simulink model "ur10_NN_v1"  (R2022b)
settings: Solver=ode4  StartTime=0.0  StopTime=5  FixedStep=0.01  MaxStep=0.1  RelTol=1e-2  AbsTol=1e-2
model workspace (MAT data in the model file):
  jointLimits = [-2.94087978961  2.94087978961; -2.50454747661  0.759218224618; -2.94087978961  2.94087978961; -2.15548162621  1.3962634016; -5.06145483078  5.06145483078; -1.53588974176  2.40855436775; -3.99680398707  3.99680398707; 0  0.025; 0  0.025; -2.94087978961  2.94087978961; -2.50454747661  0.759218224618; -2.94087978961  2.94087978961; -2.15548162621  1.3962634016; -5.06145483078  5.06145483078; -1.53588974176  2.40855436775; -3.99680398707  3.99680398707; 0  0.025; 0  0.025]
  q_points = [-0.521158884693  0.491931392418; -0.226045107026  -0.192139666701; -0.000470673510356  -0.00321781893086; 0.204187486975  0.0825184830426; -0.516935337839  0.505690245866; 0.0199734933983  0.0998802945608]
undefined symbols (not defined in the file): cbf_parms, obstacle, replay_rate, ur10
libraries: robotmaniplib x29, neural x27, robotcorelib x10
(part 1 of 2)
settings Model: PauseTimes=3.1  PacingRate=0.220000  Creator=The MathWorks, Inc.  LastModifiedBy=14244039
settings SolverCC: AlgebraicLoopSolver=TrustRegion
settings DebuggingCC: UnconnectedInputMsg=warning  UnconnectedOutputMsg=warning  UnconnectedLineMsg=warning  SFMachineParentedDataDiag=warning
settings ModelReferenceCC: EnableRefExpFcnMdlSchedulingChecks=on
settings RTWCC: DLArmComputeVersion=19.05

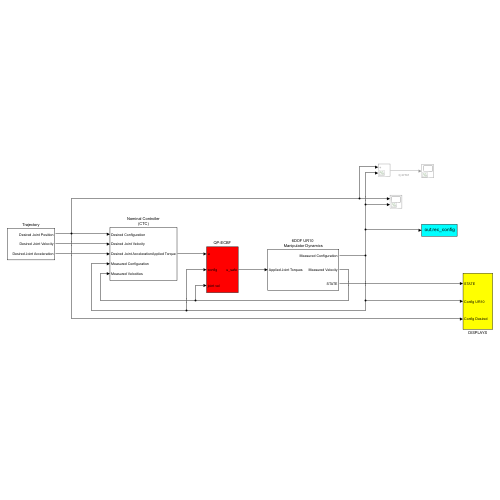
[thumbnail: Simulink's stored preview of the top-level diagram]
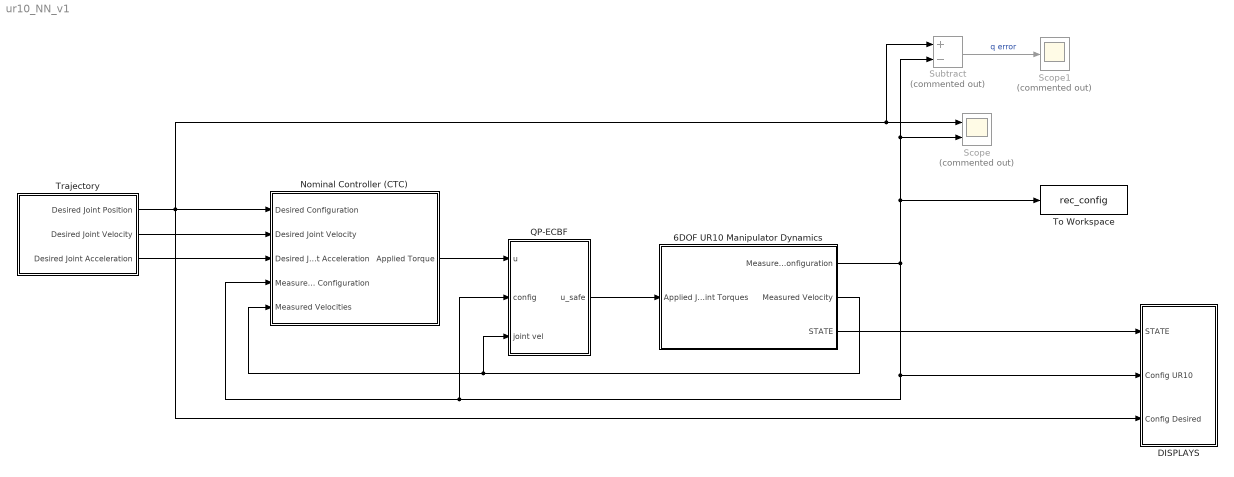
== system ur10_NN_v1 ==
  6DOF UR10 Manipulator Dynamics : Subsystem
  DISPLAYS : Subsystem
  Nominal Controller (CTC) : Subsystem
  QP-ECBF : Subsystem
  Scope : Scope  Commented=on  NumInputPorts=2
  Scope1 : Scope  Commented=on
  Subtract : Sum  Commented=on  Inputs=+-
  To Workspace : ToWorkspace  VariableName=rec_config  SampleTime=replay_rate
  Trajectory : Subsystem
  wires:
  6DOF UR10 Manipulator Dynamics/1(Measured Configuration) -> Subtract/2, Scope/2, To Workspace/1, QP-ECBF/2(config), Nominal Controller (CTC)/4(Measured Configuration), DISPLAYS/2(Config UR10)
  6DOF UR10 Manipulator Dynamics/2(Measured Velocity) -> QP-ECBF/3(joint vel), Nominal Controller (CTC)/5(Measured Velocities)
  Nominal Controller (CTC)/1(Applied Torque) -> QP-ECBF/1(u)
  Subtract/1 -> Scope1/1  "q error"
  QP-ECBF/1(u_safe) -> 6DOF UR10 Manipulator Dynamics/1(Applied Joint Torques)
  6DOF UR10 Manipulator Dynamics/3(STATE) -> DISPLAYS/1(STATE)
  Trajectory/1(Desired Joint Position) -> DISPLAYS/3(Config Desired), Subtract/1, Scope/1, Nominal Controller (CTC)/1(Desired Configuration)
  Trajectory/2(Desired Joint Velocity) -> Nominal Controller (CTC)/2(Desired Joint Velocity)
  Trajectory/3(Desired Joint Acceleration) -> Nominal Controller (CTC)/3(Desired Joint Acceleration)

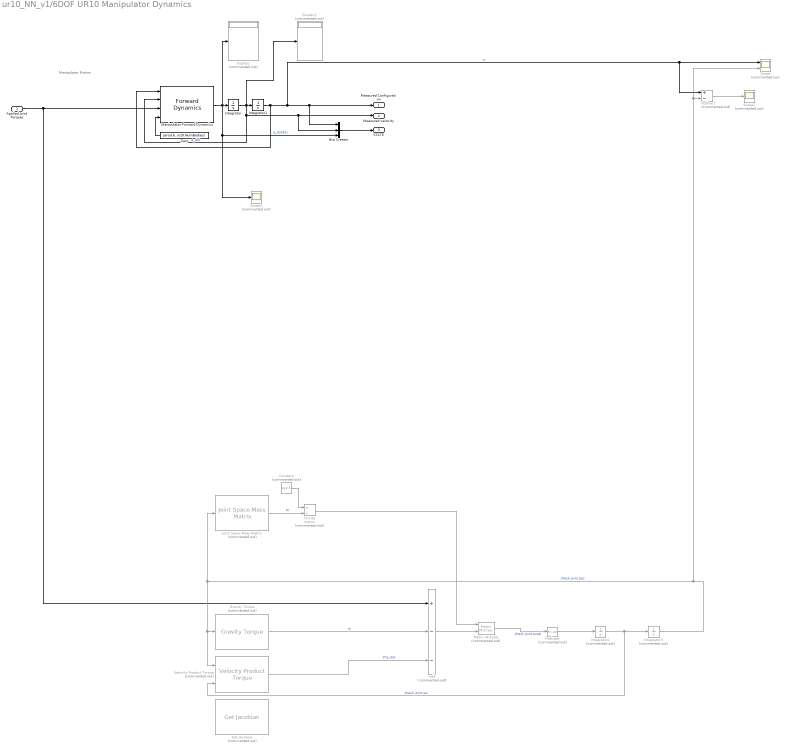
== system ur10_NN_v1/6DOF UR10 Manipulator Dynamics ==
  note: Manipulator Motion
  Applied Joint Torques : Inport
  Add : Sum  Commented=on  Inputs=+--
  Bus Creator : BusCreator  Inputs=3
  Constant : Constant  Commented=on  Value=eye(6)
  Display : Display  Commented=on
  Display1 : Display  Commented=on
  Divide : Product  Commented=on  Inputs=*/  Multiplication=Matrix(*)
  Get Jacobian : robotmaniplib/Get Jacobian  Commented=on  RigidBodyTree=ur10  EndEffector=tool0  SimulateUsing=Interpreted execution
  Gravity Torque : robotmaniplib/Gravity Torque  Commented=on  RigidBodyTree=ur10  SimulateUsing=Interpreted execution
  Integrator : Integrator  InitialCondition=[0 0 0 0 0 0]  UpperSaturationLimit=1000  LowerSaturationLimit=-1000
  Integrator1 : Integrator  InitialCondition=[0 0 0 0 0 0]  UpperSaturationLimit=jointLimits(:,2)  LowerSaturationLimit=jointLimits(:,1)
  Integrator2 : Integrator  Commented=on  InitialCondition=[0 0 0 0 0 0]'
  Integrator3 : Integrator  Commented=on  InitialCondition=[0 0 0 0 0 0]'
  Joint Space Mass Matrix : robotmaniplib/Joint Space Mass Matrix  Commented=on  RigidBodyTree=ur10  SimulateUsing=Interpreted execution
  Manipulator Forward Dynamics : robotmaniplib/Forward Dynamics  RigidBodyTree=ur10  SimulateUsing=Interpreted execution
  Matrix Multiply : Product  Commented=on  Multiplication=Matrix(*)
  Reshape : Reshape  Commented=on
  Scope : Scope  Commented=on  NumInputPorts=2
  Scope1 : Scope  Commented=on
  Scope2 : Scope  Commented=on
  Subtract : Sum  Commented=on  Inputs=+-
  Velocity Product Torque : robotmaniplib/Velocity Product Torque  Commented=on  RigidBodyTree=ur10  SimulateUsing=Interpreted execution
  Zero : Constant  Value=zeros(6, ur10.NumBodies)  OutDataTypeStr=Inherit: Inherit via back propagation
  Measured Configuration : Outport  VectorParamsAs1DForOutWhenUnconnected=off
  Measured Velocity : Outport  Port=2  VectorParamsAs1DForOutWhenUnconnected=off
  STATE : Outport  Port=3  VectorParamsAs1DForOutWhenUnconnected=off
  wires:
  Zero/1 -> Manipulator Forward Dynamics/4
  Integrator/1 -> Display1/1, Manipulator Forward Dynamics/2, Measured Velocity/1, Bus Creator/2, Integrator1/1  "q_dot"
  Applied Joint Torques/1 -> Add/1, Manipulator Forward Dynamics/3
  Integrator1/1 -> Manipulator Forward Dynamics/1, Subtract/1, Scope/1, Measured Configuration/1, Bus Creator/1  "q"
  Manipulator Forward Dynamics/1 -> Scope2/1, Bus Creator/3, Display/1, Integrator/1  "q_dotdot"
  Subtract/1 -> Scope1/1
  Integrator2/1 -> Velocity Product Torque/2, Integrator3/1  "check joint vel"
  Velocity Product Torque/1 -> Add/3  "C*q_dot"
  Gravity Torque/1 -> Add/2  "G"
  Joint Space Mass Matrix/1 -> Divide/2  "M"
  Integrator3/1 -> Subtract/2, Scope/2, Joint Space Mass Matrix/1, Gravity Torque/1, Velocity Product Torque/1  "check joint pos"
  Add/1 -> Matrix Multiply/2
  Divide/1 -> Matrix Multiply/1
  Constant/1 -> Divide/1
  Matrix Multiply/1 -> Reshape/1  "check joint accel"
  Reshape/1 -> Integrator2/1
  Bus Creator/1 -> STATE/1

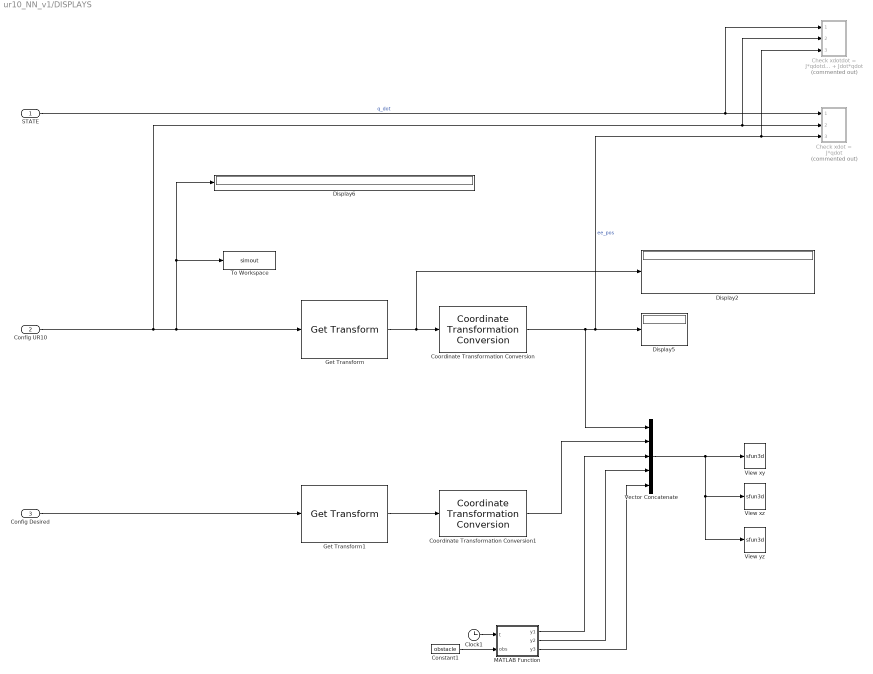
== system ur10_NN_v1/DISPLAYS ==
  STATE : Inport
  Config UR10 : Inport  Port=2
  Config Desired : Inport  Port=3
  Check xdot = J*qdot : Subsystem  Commented=on
  Check xdotdot = J*qdotdot + Jdot*qdot : Subsystem  Commented=on
  Clock1 : Clock
  Constant1 : Constant  Value=obstacle
  Coordinate Transformation Conversion : robotcorelib/Coordinate Transformation Conversion  InputRepresentation=Homogeneous Transformation  InputEulerSequence=ZYX  ShowTrVecInputPort=on  OutputRepresentation=Translation Vector  OutputEulerSequence=ZYX  ShowTrVecOutputPort=on  SimulateUsing=Interpreted execution
  Coordinate Transformation Conversion1 : robotcorelib/Coordinate Transformation Conversion  InputRepresentation=Homogeneous Transformation  InputEulerSequence=ZYX  ShowTrVecInputPort=on  OutputRepresentation=Translation Vector  OutputEulerSequence=ZYX  ShowTrVecOutputPort=on  SimulateUsing=Interpreted execution
  Display2 : Display
  Display5 : Display
  Display6 : Display
  Get Transform : robotmaniplib/Get Transform  RigidBodyTree=ur10  SourceBody=tool0  TargetBody=world  SimulateUsing=Interpreted execution
  Get Transform1 : robotmaniplib/Get Transform  RigidBodyTree=ur10  SourceBody=tool0  TargetBody=world  SimulateUsing=Interpreted execution
  MATLAB Function : MATLAB Function  TreatAsAtomicUnit=on
  To Workspace : ToWorkspace  VariableName=simout  SampleTime=-1
      settings: MaxDataPoints=1  Save2DSignal=2-D array (concatenate along first dimension)
  Vector Concatenate : Concatenate  NumInputs=5
  View xy : S-Function  LoadFcn=if exist('sfun3d','file'), sfun3d([],[],[],'LoadBlock'); end  FunctionName=sfun3d  Parameters=ax,T,np,cp,gd,ls,mk,mx,hd,tb  SFunctionDeploymentMode=off  EnableBusSupport=off  mask(3D Graph){np=5, ax=[-1.5 1.5 -1.5 1.5 -1.5 1.5], mx=1e4, T=0.1, cp=[0         0   25.9808], gd=on, hd=on, tb=on, ls=-, mk=none}
      mask prompts: np "Number of moving points (lines)"; ax "Range: [xmin xmax  ymin ymax zmin zmax]"; mx "Max number of points in each line"; T "Sampling Time"; cp "Camera position (use [0 0 1] for 2D XY view)"; gd "Grid (on|off)"; hd "HeadMarkers (on|off)"; tb "Toolbar (on|off)"; ls "LineStyle"; mk "LineMarker"
      mask help:
      | This block plots the position of several points in the XYZ space. The input contains the coordinates of all the points (x1,y1,z1,x2,y2,z2,...).
      | The number of moving points (lines), the XYZ ranges, sampling time, camera position, and grid (among other things) can be set as mask parameters.
      settings: CopyFcn=if exist('sfun3d','file'), sfun3d([],[],[],'CopyBlock'); end  DeleteFcn=if exist('sfun3d','file'), sfun3d([],[],[],'DeleteBlock'); end  NameChangeFcn=if exist('sfun3d','file'), sfun3d([],[],[],'NameChange'); end
      mask Help:
      | This block plots the position of several points in the XYZ space. The input contains the coordinates of all the points (x1,y1,z1,x2,y2,z2,...).
      | The number of moving points (lines), the XYZ ranges, sampling time, camera position, and grid (among other things) can be set as mask parameters.
      mask TypeOptions ls: - | -- | : | -. | none
      mask TypeOptions mk: none | . | + | o | * | x | square | diamond | v | ^ | > | < | pentagram | hexagram
      mask Display: plot([.05 .95 .95 .05 .05],[.45 .45 .95 .95 .45], 0.5+cos(0:0.1:2*pi)*0.3,0.7+sin(0:0.1:2*pi)*0.2)
  View xz : S-Function  LoadFcn=if exist('sfun3d','file'), sfun3d([],[],[],'LoadBlock'); end  FunctionName=sfun3d  Parameters=ax,T,np,cp,gd,ls,mk,mx,hd,tb  SFunctionDeploymentMode=off  EnableBusSupport=off  mask(3D Graph){np=5, ax=[-1.5 1.5 -1.5 1.5 -1.5 1.5], mx=1e4, T=0.1, cp=[0  -25.9808         0], gd=on, hd=on, tb=on, ls=-, mk=none}
      mask prompts: np "Number of moving points (lines)"; ax "Range: [xmin xmax  ymin ymax zmin zmax]"; mx "Max number of points in each line"; T "Sampling Time"; cp "Camera position (use [0 0 1] for 2D XY view)"; gd "Grid (on|off)"; hd "HeadMarkers (on|off)"; tb "Toolbar (on|off)"; ls "LineStyle"; mk "LineMarker"
      mask help:
      | This block plots the position of several points in the XYZ space. The input contains the coordinates of all the points (x1,y1,z1,x2,y2,z2,...).
      | The number of moving points (lines), the XYZ ranges, sampling time, camera position, and grid (among other things) can be set as mask parameters.
      settings: CopyFcn=if exist('sfun3d','file'), sfun3d([],[],[],'CopyBlock'); end  DeleteFcn=if exist('sfun3d','file'), sfun3d([],[],[],'DeleteBlock'); end  NameChangeFcn=if exist('sfun3d','file'), sfun3d([],[],[],'NameChange'); end
      mask Help:
      | This block plots the position of several points in the XYZ space. The input contains the coordinates of all the points (x1,y1,z1,x2,y2,z2,...).
      | The number of moving points (lines), the XYZ ranges, sampling time, camera position, and grid (among other things) can be set as mask parameters.
      mask TypeOptions ls: - | -- | : | -. | none
      mask TypeOptions mk: none | . | + | o | * | x | square | diamond | v | ^ | > | < | pentagram | hexagram
      mask Display: plot([.05 .95 .95 .05 .05],[.45 .45 .95 .95 .45], 0.5+cos(0:0.1:2*pi)*0.3,0.7+sin(0:0.1:2*pi)*0.2)
  View yz : S-Function  LoadFcn=if exist('sfun3d','file'), sfun3d([],[],[],'LoadBlock'); end  FunctionName=sfun3d  Parameters=ax,T,np,cp,gd,ls,mk,mx,hd,tb  SFunctionDeploymentMode=off  EnableBusSupport=off  mask(3D Graph){np=5, ax=[-1.5 1.5 -0.1 1.5 -1.5 1.5], mx=1e4, T=0.1, cp=[ 25.6976    0.8076   -0.1347], gd=on, hd=on, tb=on, ls=-, mk=none}
      mask prompts: np "Number of moving points (lines)"; ax "Range: [xmin xmax  ymin ymax zmin zmax]"; mx "Max number of points in each line"; T "Sampling Time"; cp "Camera position (use [0 0 1] for 2D XY view)"; gd "Grid (on|off)"; hd "HeadMarkers (on|off)"; tb "Toolbar (on|off)"; ls "LineStyle"; mk "LineMarker"
      mask help:
      | This block plots the position of several points in the XYZ space. The input contains the coordinates of all the points (x1,y1,z1,x2,y2,z2,...).
      | The number of moving points (lines), the XYZ ranges, sampling time, camera position, and grid (among other things) can be set as mask parameters.
      settings: CopyFcn=if exist('sfun3d','file'), sfun3d([],[],[],'CopyBlock'); end  DeleteFcn=if exist('sfun3d','file'), sfun3d([],[],[],'DeleteBlock'); end  NameChangeFcn=if exist('sfun3d','file'), sfun3d([],[],[],'NameChange'); end
      mask Help:
      | This block plots the position of several points in the XYZ space. The input contains the coordinates of all the points (x1,y1,z1,x2,y2,z2,...).
      | The number of moving points (lines), the XYZ ranges, sampling time, camera position, and grid (among other things) can be set as mask parameters.
      mask TypeOptions ls: - | -- | : | -. | none
      mask TypeOptions mk: none | . | + | o | * | x | square | diamond | v | ^ | > | < | pentagram | hexagram
      mask Display: plot([.05 .95 .95 .05 .05],[.45 .45 .95 .95 .45], 0.5+cos(0:0.1:2*pi)*0.3,0.7+sin(0:0.1:2*pi)*0.2)
  wires:
  MATLAB Function/1(y1) -> Vector Concatenate/3
  MATLAB Function/2(y2) -> Vector Concatenate/4
  Get Transform/1 -> Display2/1, Coordinate Transformation Conversion/1
  Config UR10/1 -> Check xdotdot = J*qdotdot + Jdot*qdot/2(Config), Check xdot = J*qdot/2(Config), Display6/1, To Workspace/1, Get Transform/1
  Clock1/1 -> MATLAB Function/1(t)
  MATLAB Function/3(y3) -> Vector Concatenate/5
  Config Desired/1 -> Get Transform1/1
  Vector Concatenate/1 -> View yz/1, View xz/1, View xy/1
  Coordinate Transformation Conversion/1 -> Vector Concatenate/1, Check xdotdot = J*qdotdot + Jdot*qdot/3(ee_pos), Check xdot = J*qdot/3(ee_pos), Display5/1  "ee_pos"
  Get Transform1/1 -> Coordinate Transformation Conversion1/1
  Coordinate Transformation Conversion1/1 -> Vector Concatenate/2
  STATE/1 -> Check xdotdot = J*qdotdot + Jdot*qdot/1(STATE), Check xdot = J*qdot/1(STATE)  "q_dot"
  Constant1/1 -> MATLAB Function/2(obs)

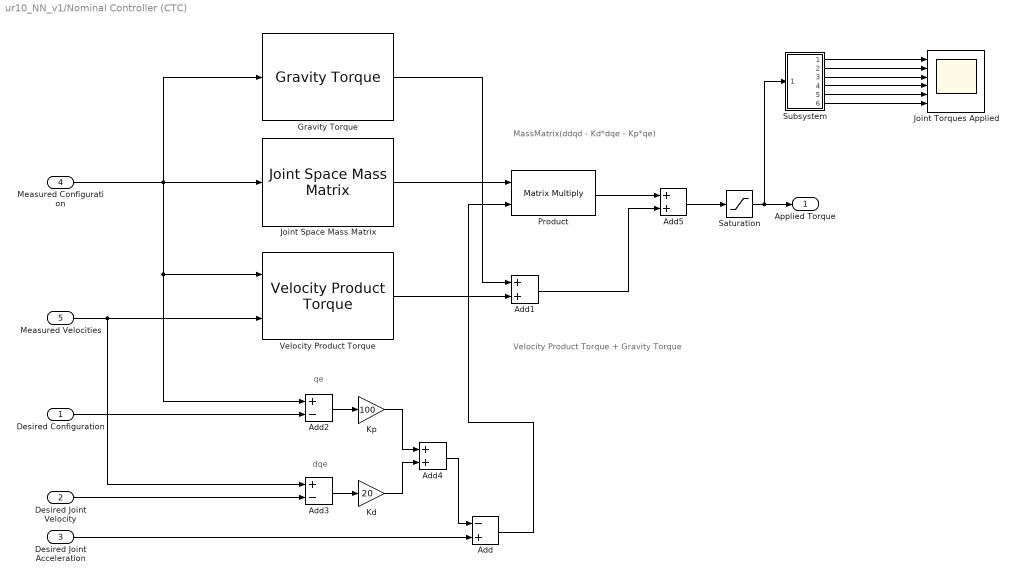
== system ur10_NN_v1/Nominal Controller (CTC) ==
  note: MassMatrix(ddqd - Kd*dqe - Kp*qe)
  note: Velocity Product Torque + Gravity Torque
  note: dqe
  note: qe
  Desired Configuration : Inport
  Desired Joint Velocity : Inport  Port=2
  Desired Joint Acceleration : Inport  Port=3
  Measured Configuration : Inport  Port=4
  Measured Velocities : Inport  Port=5
  Add : Sum  Inputs=-+
  Add1 : Sum
  Add2 : Sum  Inputs=+-
  Add3 : Sum  Inputs=+-
  Add4 : Sum
  Add5 : Sum
  Gravity Torque : robotmaniplib/Gravity Torque  RigidBodyTree=ur10  SimulateUsing=Interpreted execution
  Joint Space Mass Matrix : robotmaniplib/Joint Space Mass Matrix  RigidBodyTree=ur10  SimulateUsing=Interpreted execution
  Joint Torques Applied : Scope  NumInputPorts=6
  Kd : Gain  Gain=20
  Kp : Gain  Gain=100
  Product : Product  Multiplication=Matrix(*)
  Saturation : Saturate  UpperLimit=150  LowerLimit=-150
  Subsystem : Subsystem
  Velocity Product Torque : robotmaniplib/Velocity Product Torque  RigidBodyTree=ur10  SimulateUsing=Interpreted execution
  Applied Torque : Outport  VectorParamsAs1DForOutWhenUnconnected=off
  wires:
  Saturation/1 -> Subsystem/1(In1), Applied Torque/1
  Velocity Product Torque/1 -> Add1/2
  Add1/1 -> Add5/2
  Product/1 -> Add5/1
  Add5/1 -> Saturation/1
  Kd/1 -> Add4/2
  Kp/1 -> Add4/1
  Add3/1 -> Kd/1
  Add2/1 -> Kp/1
  Add/1 -> Product/2
  Add4/1 -> Add/1
  Measured Velocities/1 -> Velocity Product Torque/2, Add3/1
  Measured Configuration/1 -> Add2/1, Velocity Product Torque/1, Gravity Torque/1, Joint Space Mass Matrix/1
  Joint Space Mass Matrix/1 -> Product/1
  Desired Configuration/1 -> Add2/2
  Desired Joint Velocity/1 -> Add3/2
  Desired Joint Acceleration/1 -> Add/2
  Gravity Torque/1 -> Add1/1
  Subsystem/1(Out1) -> Joint Torques Applied/1
  Subsystem/2(Out2) -> Joint Torques Applied/2
  Subsystem/3(Out3) -> Joint Torques Applied/3
  Subsystem/4(Out4) -> Joint Torques Applied/4
  Subsystem/5(Out5) -> Joint Torques Applied/5
  Subsystem/6(Out6) -> Joint Torques Applied/6

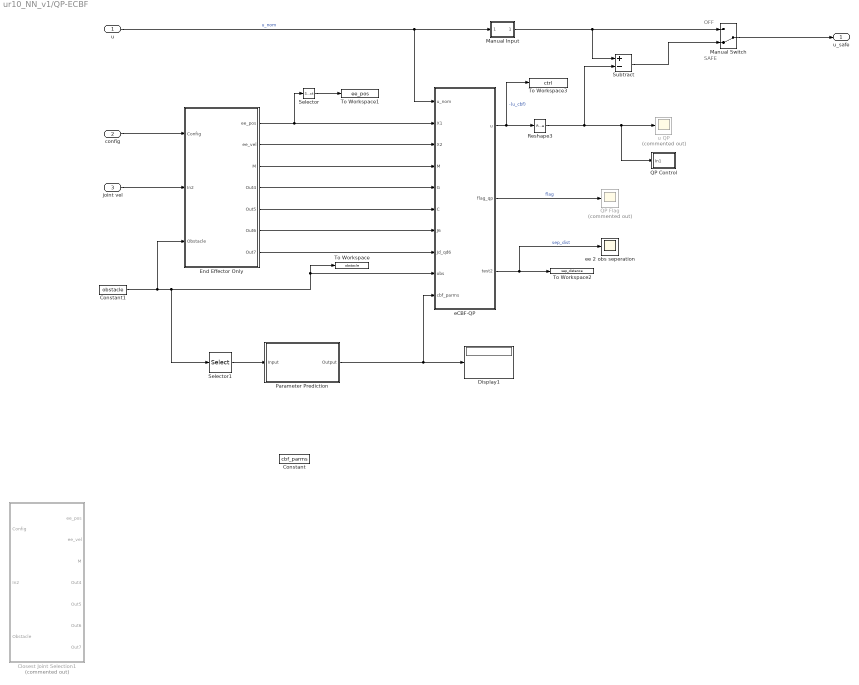
== system ur10_NN_v1/QP-ECBF ==
  note: SAFE
  note: OFF
  u : Inport
  config : Inport  Port=2
  joint vel : Inport  Port=3
  Closest Joint Selection1 : Subsystem  Commented=on
  Constant : Constant  Value=cbf_parms  VectorParams1D=off
  Constant1 : Constant  Value=obstacle
  Display1 : Display
  End Effector Only : Subsystem
  Manual Input : Subsystem
  Manual Switch : ManualSwitch  CurrentSetting=0
  Parameter Prediction : Subsystem
      mask help: Function Fitting Neural Network
      mask Display: e = 0.06;c1 = [120 150 230]/255;c2 = ([120 150 230]+0)/383;c3 = ([120 150 230]+128)/383;patch([0 1 1 0],[0 0 1 1],c1);patch([0 1 1 1-e 1-e 0+e],[0 0 1 1-e 0+e 0+e],c2);patch([0 0 1 1-e 0+e 0+e],[0 1 1 1-e 1-e 0+e],c3);plot([0 1 1 0 0],[0 0 1 1 0]);fprintf('NNET');port_label('input',1,' Input');port_label('output',1,'Output ');
  QP Control : Subsystem
  QP Flag : Scope  Commented=on
  Reshape3 : Reshape  OutputDimensionality=Column vector (2-D)
  Selector : Selector  InputPortWidth=6  IndexOptions=Index vector (dialog)  Indices=4:6  OutputSizes=1
  Selector1 : Selector  InputPortWidth=4  IndexOptions=Index vector (dialog)  Indices=4  OutputSizes=1
  Subtract : Sum  Inputs=+-
  To Workspace : ToWorkspace  VariableName=obstacle  SampleTime=-1
      settings: MaxDataPoints=1
  To Workspace1 : ToWorkspace  VariableName=ee_pos  SampleTime=replay_rate
  To Workspace2 : ToWorkspace  VariableName=sep_distance  SampleTime=replay_rate
  To Workspace3 : ToWorkspace  VariableName=ctrl  SampleTime=replay_rate
  eCBF-QP : MATLAB Function  TreatAsAtomicUnit=on
  ee 2 obs seperation : Scope
  u QP : Scope  Commented=on
  u_safe : Outport
  wires:
  u/1 -> Manual Input/1(u_nom), eCBF-QP/1(u_nom)  "u_nom"
  Manual Switch/1 -> u_safe/1
  Constant1/1 -> End Effector Only/3(Obstacle), Selector1/1, eCBF-QP/9(obs), To Workspace/1
  eCBF-QP/1(u) -> To Workspace3/1, Reshape3/1  "-(u_cbf)"
  Subtract/1 -> Manual Switch/2
  Reshape3/1 -> Subtract/2, QP Control/1(In1), u QP/1
  eCBF-QP/3(test2) -> ee 2 obs seperation/1, To Workspace2/1  "sep_dist"
  config/1 -> End Effector Only/1(Config)
  End Effector Only/1(ee_pos) -> Selector/1, eCBF-QP/2(X1)
  End Effector Only/2(ee_vel) -> eCBF-QP/3(X2)
  End Effector Only/3(M) -> eCBF-QP/4(M)
  End Effector Only/4(Out4) -> eCBF-QP/5(G)
  End Effector Only/5(Out5) -> eCBF-QP/6(C)
  End Effector Only/6(Out6) -> eCBF-QP/7(J6)
  End Effector Only/7(Out7) -> eCBF-QP/8(Jd_qd6)
  joint vel/1 -> End Effector Only/2(In2)
  eCBF-QP/2(flag_qp) -> QP Flag/1  "flag"
  Manual Input/1(Out1) -> Manual Switch/1, Subtract/1
  Selector/1 -> To Workspace1/1
  Selector1/1 -> Parameter Prediction/1(Input)
  Parameter Prediction/1(Output) -> eCBF-QP/10(cbf_parms), Display1/1

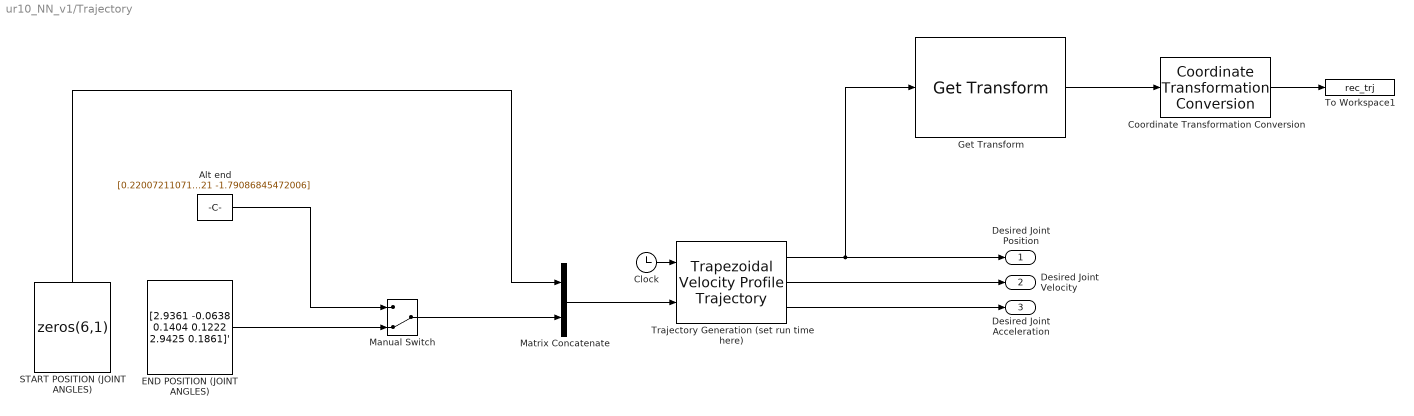
== system ur10_NN_v1/Trajectory ==
  Alt end : Constant  Value=|  VectorParams1D=off
      | [0.220072110712972
      | -2.20878169107432
      | -1.50641761454312
      | 2.14440297377872
      | 1.57079633561621
      | -1.79086845472006]
  Clock : Clock
  Coordinate Transformation Conversion : robotcorelib/Coordinate Transformation Conversion  InputRepresentation=Homogeneous Transformation  InputEulerSequence=ZYX  ShowTrVecInputPort=on  OutputRepresentation=Translation Vector  OutputEulerSequence=ZYX  ShowTrVecOutputPort=on  SimulateUsing=Interpreted execution
  END POSITION (JOINT ANGLES) : Constant  Value=[2.9361 -0.0638 0.1404 0.1222 2.9425 0.1861]'  VectorParams1D=off
  Get Transform : robotmaniplib/Get Transform  RigidBodyTree=ur10  SourceBody=tool0  TargetBody=world  SimulateUsing=Interpreted execution
  Manual Switch : ManualSwitch  CurrentSetting=0
  Matrix Concatenate : Concatenate  Mode=Multidimensional array  ConcatenateDimension=2
  START POSITION (JOINT ANGLES) : Constant  Value=zeros(6,1)  VectorParams1D=off
  To Workspace1 : ToWorkspace  VariableName=rec_trj  SampleTime=replay_rate
  Trajectory Generation (set run time here) : robotcorelib/Trapezoidal Velocity Profile Trajectory  WaypointSource=External  Waypoints=[ 0, -0.5, -1; 0, 0.5, 1 ]  NumParams=1  Parameter1=End Time  Parameter2=End Time  ParameterSource=Internal  PeakVelocity=[ 2; 2 ]  Acceleration=[ 1; 2 ]  EndTime=5  AccelTime=[ 1; 2 ]  SimulateUsing=Interpreted execution
  Desired Joint Position : Outport
  Desired Joint Velocity : Outport  Port=2
  Desired Joint Acceleration : Outport  Port=3
  wires:
  Alt end/1 -> Manual Switch/1
  Trajectory Generation (set run time here)/1 -> Desired Joint Position/1, Get Transform/1
  Get Transform/1 -> Coordinate Transformation Conversion/1
  Clock/1 -> Trajectory Generation (set run time here)/1
  START POSITION (JOINT ANGLES)/1 -> Matrix Concatenate/1
  Matrix Concatenate/1 -> Trajectory Generation (set run time here)/2
  Manual Switch/1 -> Matrix Concatenate/2
  END POSITION (JOINT ANGLES)/1 -> Manual Switch/2
  Coordinate Transformation Conversion/1 -> To Workspace1/1
  Trajectory Generation (set run time here)/2 -> Desired Joint Velocity/1
  Trajectory Generation (set run time here)/3 -> Desired Joint Acceleration/1

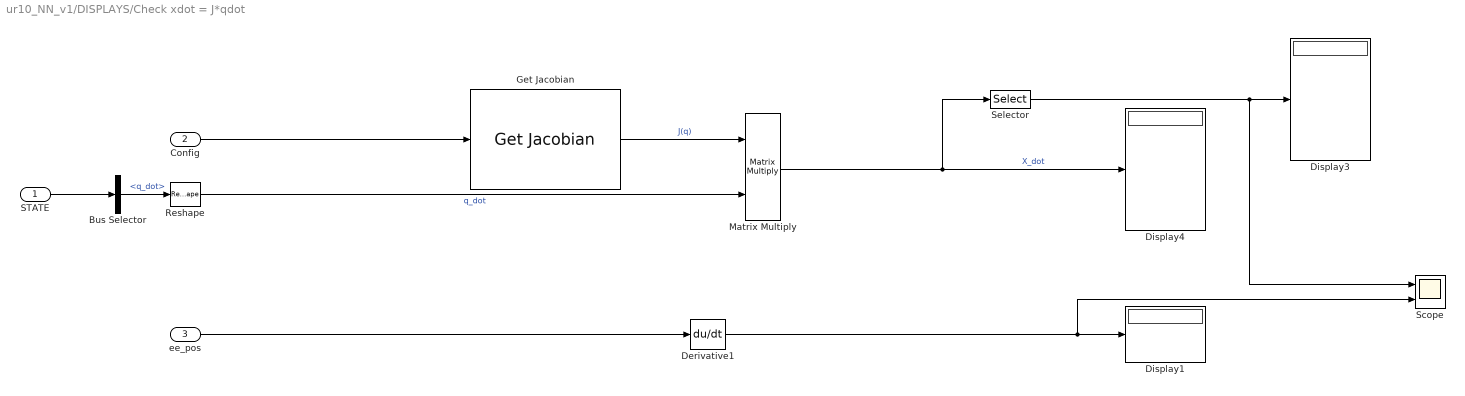
== system ur10_NN_v1/DISPLAYS/Check xdot = J*qdot ==
  STATE : Inport
  Config : Inport  Port=2
  ee_pos : Inport  Port=3
  Bus Selector : BusSelector  OutputSignals=q_dot
  Derivative1 : Derivative
  Display1 : Display
  Display3 : Display
  Display4 : Display
  Get Jacobian : robotmaniplib/Get Jacobian  RigidBodyTree=ur10  EndEffector=tool0  SimulateUsing=Interpreted execution
  Matrix Multiply : Product  Multiplication=Matrix(*)
  Reshape : Reshape  OutputDimensionality=Column vector (2-D)
  Scope : Scope  NumInputPorts=2
  Selector : Selector  InputPortWidth=6  IndexOptions=Index vector (dialog)  Indices=4:6  OutputSizes=1
  wires:
  Selector/1 -> Scope/1, Display3/1
  Config/1 -> Get Jacobian/1
  Derivative1/1 -> Scope/2, Display1/1
  STATE/1 -> Bus Selector/1
  Get Jacobian/1 -> Matrix Multiply/1  "J(q)"
  Matrix Multiply/1 -> Selector/1, Display4/1  "X_dot"
  ee_pos/1 -> Derivative1/1
  Bus Selector/1 -> Reshape/1  "<q_dot>"
  Reshape/1 -> Matrix Multiply/2  "q_dot"

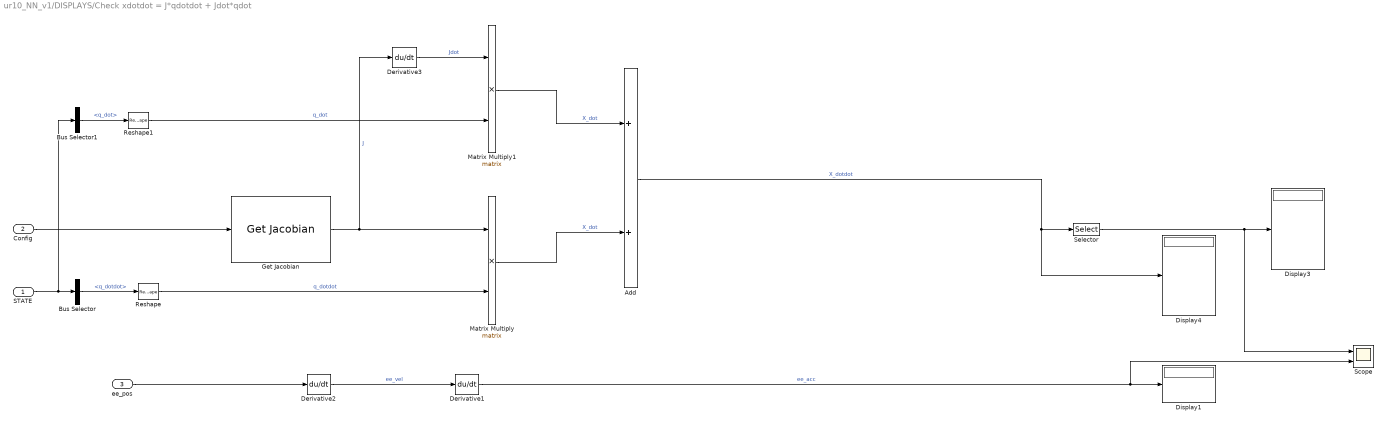
== system ur10_NN_v1/DISPLAYS/Check xdotdot = J*qdotdot + Jdot*qdot ==
  STATE : Inport
  Config : Inport  Port=2
  ee_pos : Inport  Port=3
  Add : Sum
  Bus Selector : BusSelector  OutputSignals=q_dotdot
  Bus Selector1 : BusSelector  OutputSignals=q_dot
  Derivative1 : Derivative
  Derivative2 : Derivative
  Derivative3 : Derivative
  Display1 : Display
  Display3 : Display
  Display4 : Display
  Get Jacobian : robotmaniplib/Get Jacobian  RigidBodyTree=ur10  EndEffector=tool0  SimulateUsing=Interpreted execution
  Matrix Multiply : Product  Multiplication=Matrix(*)
  Matrix Multiply1 : Product  Multiplication=Matrix(*)
  Reshape : Reshape  OutputDimensionality=Column vector (2-D)
  Reshape1 : Reshape  OutputDimensionality=Column vector (2-D)
  Scope : Scope  NumInputPorts=2
  Selector : Selector  InputPortWidth=6  IndexOptions=Index vector (dialog)  Indices=4:6  OutputSizes=1
  wires:
  Reshape/1 -> Matrix Multiply/2  "q_dotdot"
  Bus Selector/1 -> Reshape/1  "<q_dotdot>"
  ee_pos/1 -> Derivative2/1
  Add/1 -> Display4/1, Selector/1  "X_dotdot"
  Get Jacobian/1 -> Matrix Multiply/1, Derivative3/1  "J"
  STATE/1 -> Bus Selector1/1, Bus Selector/1
  Derivative1/1 -> Display1/1, Scope/2  "ee_acc"
  Config/1 -> Get Jacobian/1
  Selector/1 -> Display3/1, Scope/1
  Derivative2/1 -> Derivative1/1  "ee_vel"
  Derivative3/1 -> Matrix Multiply1/1  "Jdot"
  Bus Selector1/1 -> Reshape1/1  "<q_dot>"
  Reshape1/1 -> Matrix Multiply1/2  "q_dot"
  Matrix Multiply1/1 -> Add/1  "X_dot"
  Matrix Multiply/1 -> Add/2  "X_dot"

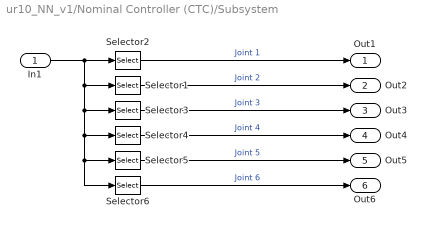
== system ur10_NN_v1/Nominal Controller (CTC)/Subsystem ==
  In1 : Inport
  Selector1 : Selector  InputPortWidth=6  IndexOptions=Index vector (dialog)  Indices=2  OutputSizes=1
  Selector2 : Selector  InputPortWidth=6  IndexOptions=Index vector (dialog)  Indices=1  OutputSizes=1
  Selector3 : Selector  InputPortWidth=6  IndexOptions=Index vector (dialog)  Indices=3  OutputSizes=1
  Selector4 : Selector  InputPortWidth=6  IndexOptions=Index vector (dialog)  Indices=4  OutputSizes=1
  Selector5 : Selector  InputPortWidth=6  IndexOptions=Index vector (dialog)  Indices=5  OutputSizes=1
  Selector6 : Selector  InputPortWidth=6  IndexOptions=Index vector (dialog)  Indices=6  OutputSizes=1
  Out1 : Outport
  Out2 : Outport  Port=2
  Out3 : Outport  Port=3
  Out4 : Outport  Port=4
  Out5 : Outport  Port=5
  Out6 : Outport  Port=6
  wires:
  In1/1 -> Selector2/1, Selector3/1, Selector4/1, Selector5/1, Selector6/1, Selector1/1
  Selector2/1 -> Out1/1  "Joint 1"
  Selector1/1 -> Out2/1  "Joint 2"
  Selector3/1 -> Out3/1  "Joint 3"
  Selector4/1 -> Out4/1  "Joint 4"
  Selector5/1 -> Out5/1  "Joint 5"
  Selector6/1 -> Out6/1  "Joint 6"

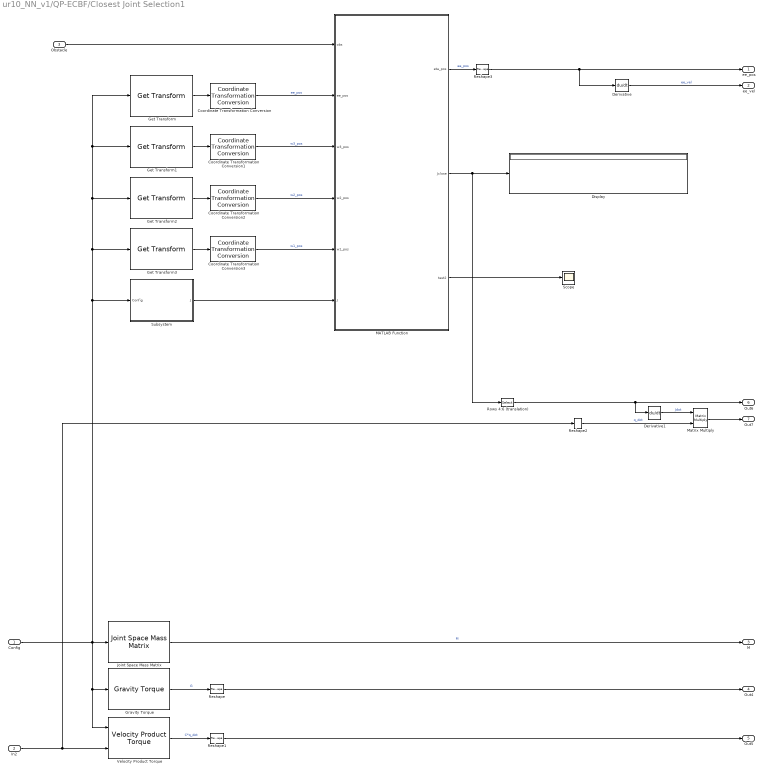
== system ur10_NN_v1/QP-ECBF/Closest Joint Selection1 ==
  Config : Inport
  In2 : Inport  Port=2
  Obstacle : Inport  Port=3
  Coordinate Transformation Conversion{,1..3} (4 alike) : robotcorelib/Coordinate Transformation Conversion  InputRepresentation=Homogeneous Transformation  InputEulerSequence=ZYX  ShowTrVecInputPort=on  OutputRepresentation=Translation Vector  OutputEulerSequence=ZYX  ShowTrVecOutputPort=on  SimulateUsing=Interpreted execution
  Derivative : Derivative
  Derivative1 : Derivative
  Display : Display
  Get Transform : robotmaniplib/Get Transform  RigidBodyTree=ur10  SourceBody=tool0  TargetBody=world  SimulateUsing=Interpreted execution
  Get Transform1 : robotmaniplib/Get Transform  RigidBodyTree=ur10  SourceBody=wrist_3_link  TargetBody=world  SimulateUsing=Interpreted execution
  Get Transform2 : robotmaniplib/Get Transform  RigidBodyTree=ur10  SourceBody=wrist_2_link  TargetBody=world  SimulateUsing=Interpreted execution
  Get Transform3 : robotmaniplib/Get Transform  RigidBodyTree=ur10  SourceBody=wrist_1_link  TargetBody=world  SimulateUsing=Interpreted execution
  Gravity Torque : robotmaniplib/Gravity Torque  RigidBodyTree=ur10  SimulateUsing=Interpreted execution
  Joint Space Mass Matrix : robotmaniplib/Joint Space Mass Matrix  RigidBodyTree=ur10  SimulateUsing=Interpreted execution
  MATLAB Function : MATLAB Function  TreatAsAtomicUnit=on
  Matrix Multiply : Product  Multiplication=Matrix(*)
  Reshape{,1..3} (4 alike) : Reshape  OutputDimensionality=Column vector (2-D)
  Rows 4:6 (translation) : Selector  NumberOfDimensions=2  InputPortWidth=3  IndexOptions=Index vector (dialog),Index vector (dialog)  Indices=4:6,1:6  OutputSizes=1,1
  Scope : Scope
  Subsystem : Subsystem
  Velocity Product Torque : robotmaniplib/Velocity Product Torque  RigidBodyTree=ur10  SimulateUsing=Interpreted execution
  ee_pos : Outport
  ee_vel : Outport  Port=2
  M : Outport  Port=3
  Out4 : Outport  Port=4
  Out5 : Outport  Port=5
  Out6 : Outport  Port=6
  Out7 : Outport  Port=7
  wires:
  MATLAB Function/3(test2) -> Scope/1
  Reshape3/1 -> Derivative/1, ee_pos/1
  MATLAB Function/2(Jclose) -> Display/1, Rows 4:6 (translation)/1
  Subsystem/1(J) -> MATLAB Function/6(J)
  Obstacle/1 -> MATLAB Function/1(obs)
  Coordinate Transformation Conversion3/1 -> MATLAB Function/5(w1_pos)  "w1_pos"
  Coordinate Transformation Conversion2/1 -> MATLAB Function/4(w2_pos)  "w2_pos"
  Get Transform3/1 -> Coordinate Transformation Conversion3/1
  Coordinate Transformation Conversion1/1 -> MATLAB Function/3(w3_pos)  "w3_pos"
  Coordinate Transformation Conversion/1 -> MATLAB Function/2(ee_pos)  "ee_pos"
  Get Transform2/1 -> Coordinate Transformation Conversion2/1
  Get Transform1/1 -> Coordinate Transformation Conversion1/1
  Derivative/1 -> ee_vel/1  "ee_vel"
  Derivative1/1 -> Matrix Multiply/1  "Jdot"
  Matrix Multiply/1 -> Out7/1
  Rows 4:6 (translation)/1 -> Derivative1/1, Out6/1
  Reshape2/1 -> Matrix Multiply/2  "q_dot"
  Get Transform/1 -> Coordinate Transformation Conversion/1
  Reshape1/1 -> Out5/1
  Reshape/1 -> Out4/1
  MATLAB Function/1(eta_pos) -> Reshape3/1  "ee_pos"
  Joint Space Mass Matrix/1 -> M/1  "M"
  Gravity Torque/1 -> Reshape/1  "G"
  In2/1 -> Velocity Product Torque/2, Reshape2/1
  Config/1 -> Joint Space Mass Matrix/1, Gravity Torque/1, Velocity Product Torque/1, Get Transform1/1, Get Transform/1, Get Transform2/1, Get Transform3/1, Subsystem/1(Config)
  Velocity Product Torque/1 -> Reshape1/1  "C*q_dot"

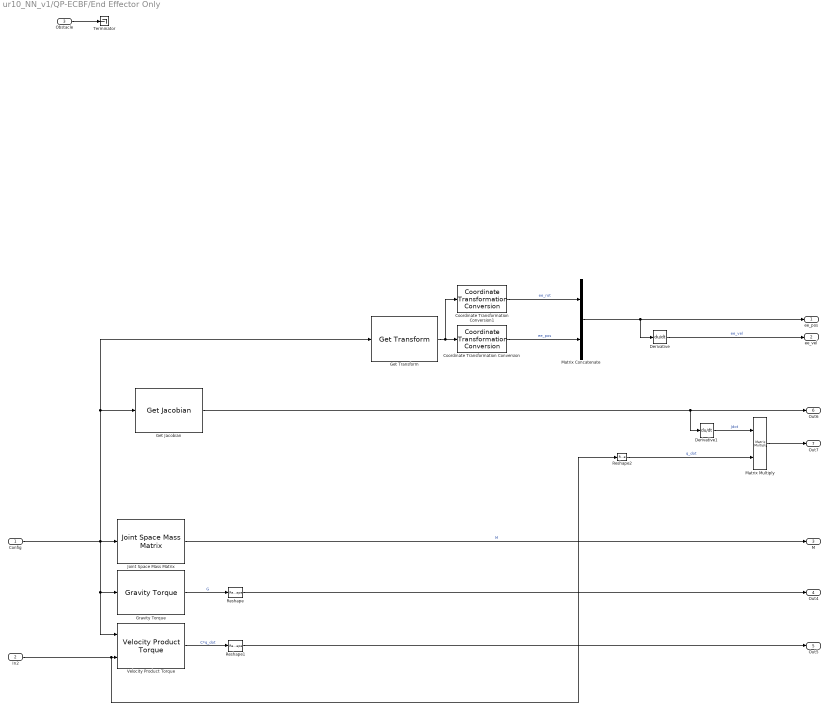
== system ur10_NN_v1/QP-ECBF/End Effector Only ==
  Config : Inport
  In2 : Inport  Port=2
  Obstacle : Inport  Port=3
  Coordinate Transformation Conversion : robotcorelib/Coordinate Transformation Conversion  InputRepresentation=Homogeneous Transformation  InputEulerSequence=ZYX  ShowTrVecInputPort=on  OutputRepresentation=Translation Vector  OutputEulerSequence=ZYX  ShowTrVecOutputPort=on  SimulateUsing=Interpreted execution
  Coordinate Transformation Conversion1 : robotcorelib/Coordinate Transformation Conversion  InputRepresentation=Homogeneous Transformation  InputEulerSequence=XYZ  ShowTrVecInputPort=on  OutputRepresentation=Euler Angles  OutputEulerSequence=XYZ  ShowTrVecOutputPort=off  SimulateUsing=Interpreted execution
  Derivative : Derivative
  Derivative1 : Derivative
  Get Jacobian : robotmaniplib/Get Jacobian  RigidBodyTree=ur10  EndEffector=tool0  SimulateUsing=Interpreted execution
  Get Transform : robotmaniplib/Get Transform  RigidBodyTree=ur10  SourceBody=tool0  TargetBody=world  SimulateUsing=Interpreted execution
  Gravity Torque : robotmaniplib/Gravity Torque  RigidBodyTree=ur10  SimulateUsing=Interpreted execution
  Joint Space Mass Matrix : robotmaniplib/Joint Space Mass Matrix  RigidBodyTree=ur10  SimulateUsing=Interpreted execution
  Matrix Concatenate : Concatenate  Mode=Multidimensional array
  Matrix Multiply : Product  Multiplication=Matrix(*)
  Reshape : Reshape  OutputDimensionality=Column vector (2-D)
  Reshape1 : Reshape  OutputDimensionality=Column vector (2-D)
  Reshape2 : Reshape  OutputDimensionality=Column vector (2-D)
  Terminator : Terminator
  Velocity Product Torque : robotmaniplib/Velocity Product Torque  RigidBodyTree=ur10  SimulateUsing=Interpreted execution
  ee_pos : Outport
  ee_vel : Outport  Port=2
  M : Outport  Port=3
  Out4 : Outport  Port=4
  Out5 : Outport  Port=5
  Out6 : Outport  Port=6
  Out7 : Outport  Port=7
  wires:
  Velocity Product Torque/1 -> Reshape1/1  "C*q_dot"
  Config/1 -> Get Transform/1, Get Jacobian/1, Velocity Product Torque/1, Gravity Torque/1, Joint Space Mass Matrix/1
  In2/1 -> Reshape2/1, Velocity Product Torque/2
  Gravity Torque/1 -> Reshape/1  "G"
  Joint Space Mass Matrix/1 -> M/1  "M"
  Reshape/1 -> Out4/1
  Reshape1/1 -> Out5/1
  Get Transform/1 -> Coordinate Transformation Conversion1/1, Coordinate Transformation Conversion/1
  Reshape2/1 -> Matrix Multiply/2  "q_dot"
  Matrix Multiply/1 -> Out7/1
  Derivative1/1 -> Matrix Multiply/1  "Jdot"
  Derivative/1 -> ee_vel/1  "ee_vel"
  Coordinate Transformation Conversion/1 -> Matrix Concatenate/2  "ee_pos"
  Obstacle/1 -> Terminator/1
  Coordinate Transformation Conversion1/1 -> Matrix Concatenate/1  "ee_rot"
  Matrix Concatenate/1 -> Derivative/1, ee_pos/1
  Get Jacobian/1 -> Out6/1, Derivative1/1

== system ur10_NN_v1/QP-ECBF/Manual Input ==
  note: u1 = shoulder link ( big base)
  note: u2 = upper arm link
  note: u3 = forearm link (mid)
  note: u4 = wrist1 link
  note: u5 = wrist 2 link
  note: u6 = wrist 3 link
  u_nom : Inport
  Constant : Constant  Value=[0 0 0 0 0 1]'  VectorParams1D=off
  Gain1 : Gain  Gain=-0.005
  Manual Switch : ManualSwitch  CurrentSetting=0
  Scope : Scope
  Out1 : Outport
  wires:
  u_nom/1 -> Manual Switch/2
  Manual Switch/1 -> Out1/1
  Constant/1 -> Gain1/1
  Gain1/1 -> Scope/1, Manual Switch/1

== system ur10_NN_v1/QP-ECBF/Parameter Prediction ==
  Input : Inport  PortDimensions=1
      mask Display: e = 0.06;c1 = [120 230 180]/255;c2 = ([120 230 180]+0)/(256+128);c3 = ([120 230 180]+128)/(256+128);patch([0 1 1 0],[0 0 1 1],c1);patch([0 1 1 1-e 1-e 0+e],[0 0 1 1-e 0+e 0+e],c2);patch([0 0 1 1-e 0+e 0+e],[0 1 1 1-e 1-e 0+e],c3);plot([0 1 1 0 0],[0 0 1 1 0]);
  Layer 1 : Subsystem
      mask Display: e = 0.06;c1 = [120 150 230]/255;c2 = ([120 150 230]+0)/383;c3 = ([120 150 230]+128)/383;patch([0 1 1 0],[0 0 1 1],c1);patch([0 1 1 1-e 1-e 0+e],[0 0 1 1-e 0+e 0+e],c2);patch([0 0 1 1-e 0+e 0+e],[0 1 1 1-e 1-e 0+e],c3);plot([0 1 1 0 0],[0 0 1 1 0]);
  Layer 2 : Subsystem
      mask Display: e = 0.06;c1 = [120 150 230]/255;c2 = ([120 150 230]+0)/383;c3 = ([120 150 230]+128)/383;patch([0 1 1 0],[0 0 1 1],c1);patch([0 1 1 1-e 1-e 0+e],[0 0 1 1-e 0+e 0+e],c2);patch([0 0 1 1-e 0+e 0+e],[0 1 1 1-e 1-e 0+e],c3);plot([0 1 1 0 0],[0 0 1 1 0]);
  Process Input 1 : Subsystem
      mask Display: e = 0.06;c1 = [120 150 230]/255;c2 = ([120 150 230]+0)/383;c3 = ([120 150 230]+128)/383;patch([0 1 1 0],[0 0 1 1],c1);patch([0 1 1 1-e 1-e 0+e],[0 0 1 1-e 0+e 0+e],c2);patch([0 0 1 1-e 0+e 0+e],[0 1 1 1-e 1-e 0+e],c3);plot([0 1 1 0 0],[0 0 1 1 0]);
  Process Output 1 : Subsystem
      mask Display: e = 0.06;c1 = [120 150 230]/255;c2 = ([120 150 230]+0)/383;c3 = ([120 150 230]+128)/383;patch([0 1 1 0],[0 0 1 1],c1);patch([0 1 1 1-e 1-e 0+e],[0 0 1 1-e 0+e 0+e],c2);patch([0 0 1 1-e 0+e 0+e],[0 1 1 1-e 1-e 0+e],c3);plot([0 1 1 0 0],[0 0 1 1 0]);
  Output : Outport  InitialOutput=[0;0;0]
      mask Display: e = 0.06;c1 = [120 230 180]/255;c2 = ([120 230 180]+0)/(256+128);c3 = ([120 230 180]+128)/(256+128);patch([0 1 1 0],[0 0 1 1],c1);patch([0 1 1 1-e 1-e 0+e],[0 0 1 1-e 0+e 0+e],c2);patch([0 0 1 1-e 0+e 0+e],[0 1 1 1-e 1-e 0+e],c3);plot([0 1 1 0 0],[0 0 1 1 0]);
  wires:
  Input/1 -> Process Input 1/1(x)
  Process Output 1/1(y) -> Output/1
  Process Input 1/1(p) -> Layer 1/1("p{1}")
  Layer 1/1("a{1}") -> [feedback1]
  [feedback1] -> Layer 2/1("a{1} ")
  Layer 2/1("a{2}") -> Process Output 1/1(a)

== system ur10_NN_v1/QP-ECBF/QP Control ==
  In1 : Inport
  CBF-QP Joint Control : Scope  NumInputPorts=6
  Selector : Selector  InputPortWidth=6  IndexOptions=Index vector (dialog)  Indices=1  OutputSizes=1
  Selector1 : Selector  InputPortWidth=6  IndexOptions=Index vector (dialog)  Indices=2  OutputSizes=1
  Selector2 : Selector  InputPortWidth=6  IndexOptions=Index vector (dialog)  Indices=3  OutputSizes=1
  Selector3 : Selector  InputPortWidth=6  IndexOptions=Index vector (dialog)  Indices=4  OutputSizes=1
  Selector4 : Selector  InputPortWidth=6  IndexOptions=Index vector (dialog)  Indices=5  OutputSizes=1
  Selector5 : Selector  InputPortWidth=6  IndexOptions=Index vector (dialog)  Indices=6  OutputSizes=1
  wires:
  In1/1 -> Selector/1, Selector1/1, Selector2/1, Selector3/1, Selector4/1, Selector5/1
  Selector/1 -> CBF-QP Joint Control/1  "joint 1 (base)"
  Selector1/1 -> CBF-QP Joint Control/2  "joint 2 (shoulder)"
  Selector2/1 -> CBF-QP Joint Control/3  "joint 3 (elbow)"
  Selector3/1 -> CBF-QP Joint Control/4  "joint 4 (wrist 1)"
  Selector4/1 -> CBF-QP Joint Control/5  "joint 5 (wrist 2)"
  Selector5/1 -> CBF-QP Joint Control/6  "joint 6 (wrist 3 ee)"

== system ur10_NN_v1/QP-ECBF/Closest Joint Selection1/Subsystem ==
  Config : Inport
  Get Jacobian : robotmaniplib/Get Jacobian  RigidBodyTree=ur10  EndEffector=tool0  SimulateUsing=Interpreted execution
  Get Jacobian1 : robotmaniplib/Get Jacobian  RigidBodyTree=ur10  EndEffector=wrist_3_link  SimulateUsing=Interpreted execution
  Get Jacobian2 : robotmaniplib/Get Jacobian  RigidBodyTree=ur10  EndEffector=wrist_2_link  SimulateUsing=Interpreted execution
  Get Jacobian3 : robotmaniplib/Get Jacobian  RigidBodyTree=ur10  EndEffector=wrist_1_link  SimulateUsing=Interpreted execution
  Matrix Concatenate : Concatenate  NumInputs=4  Mode=Multidimensional array  ConcatenateDimension=3
  J : Outport
  wires:
  Matrix Concatenate/1 -> J/1
  Get Jacobian3/1 -> Matrix Concatenate/4  "Jw1"
  Get Jacobian2/1 -> Matrix Concatenate/3  "Jw2"
  Get Jacobian1/1 -> Matrix Concatenate/2  "Jw3"
  Config/1 -> Get Jacobian/1, Get Jacobian1/1, Get Jacobian2/1, Get Jacobian3/1
  Get Jacobian/1 -> Matrix Concatenate/1  "Jee"

== system ur10_NN_v1/QP-ECBF/Parameter Prediction/Layer 1 ==
  "p{1}" : Inport  PortDimensions=1
      mask Display: e = 0.06;c1 = [120 230 180]/255;c2 = ([120 230 180]+0)/(256+128);c3 = ([120 230 180]+128)/(256+128);patch([0 1 1 0],[0 0 1 1],c1);patch([0 1 1 1-e 1-e 0+e],[0 0 1 1-e 0+e 0+e],c2);patch([0 0 1 1-e 0+e 0+e],[0 1 1 1-e 1-e 0+e],c3);plot([0 1 1 0 0],[0 0 1 1 0]);
  Delays 1 : Subsystem
      mask Display: e = 0.06;c1 = [120 150 230]/255;c2 = ([120 150 230]+0)/383;c3 = ([120 150 230]+128)/383;patch([0 1 1 0],[0 0 1 1],c1);patch([0 1 1 1-e 1-e 0+e],[0 0 1 1-e 0+e 0+e],c2);patch([0 0 1 1-e 0+e 0+e],[0 1 1 1-e 1-e 0+e],c3);plot([0 1 1 0 0],[0 0 1 1 0]);disp('0');
  "IW{1,1}" : Subsystem
      mask Display: e = 0.06;c1 = [120 150 230]/255;c2 = ([120 150 230]+0)/383;c3 = ([120 150 230]+128)/383;patch([0 1 1 0],[0 0 1 1],c1);patch([0 1 1 1-e 1-e 0+e],[0 0 1 1-e 0+e 0+e],c2);patch([0 0 1 1-e 0+e 0+e],[0 1 1 1-e 1-e 0+e],c3);plot([0 1 1 0 0],[0 0 1 1 0]);disp('W');
  "b{1}" : Constant  Value=[-0.4817697371321660870790992703405208885669708251953125;-0.404346948350879475952979191788472235202789306640625;0.374556355738183188730516803843784146010875701904296875;-0.303418659356770648027890047160326503217220306396484375;-0.24500020941144295960611998452804982662200927734375;0.2146363159208510840159078725264407694339752197265625;0.1744985749533798091714942302132840268313884735107421875;-0.120584494229239502782746740194852463901042938232421875;-0.076503223353235838555264081151108257472515106201171875;-0.0219681027123705720216495507202125736512243747711181640625;-0.028149194962190239588384343960569822229444980621337890625;0.0751813974618122937698672103579156100749969482421875;0.1199333067596103086227543599306955002248287200927734375;-0.1602507066613770569940555787979974411427974700927734375;0.207463426395334937790693174974876455962657928466796875;-0.248529508503928575624541963406954891979694366455078125;-0.308016601913519760813642278662882745265960693359375;0.3525289101667485880398089648224413394927978515625;0.39578251632452232655623447499237954616546630859375;0.44153833971519507173297824920155107975006103515625]
      mask Display: e = 0.06;c1 = [120 150 230]/255;c2 = ([120 150 230]+0)/383;c3 = ([120 150 230]+128)/383;patch([0 1 1 0],[0 0 1 1],c1);patch([0 1 1 1-e 1-e 0+e],[0 0 1 1-e 0+e 0+e],c2);patch([0 0 1 1-e 0+e 0+e],[0 1 1 1-e 1-e 0+e],c3);plot([0 1 1 0 0],[0 0 1 1 0]);disp('b');
  netsum : Sum  Inputs=2  InputSameDT=on  SaturateOnIntegerOverflow=on  OutDataTypeStr=Inherit: Same as first input
      mask Display: e = 0.06;c1 = [120 150 230]/255;c2 = ([120 150 230]+0)/383;c3 = ([120 150 230]+128)/383;patch([0 1 1 0],[0 0 1 1],c1);patch([0 1 1 1-e 1-e 0+e],[0 0 1 1-e 0+e 0+e],c2);patch([0 0 1 1-e 0+e 0+e],[0 1 1 1-e 1-e 0+e],c3);plot([0 1 1 0 0],[0 0 1 1 0]);disp('+');
  tansig : neural/Transfer Functions/tansig
  "a{1}" : Outport  InitialOutput=[0;0;0;0;0;0;0;0;0;0;0;0;0;0;0;0;0;0;0;0]
      mask Display: e = 0.06;c1 = [120 230 180]/255;c2 = ([120 230 180]+0)/(256+128);c3 = ([120 230 180]+128)/(256+128);patch([0 1 1 0],[0 0 1 1],c1);patch([0 1 1 1-e 1-e 0+e],[0 0 1 1-e 0+e 0+e],c2);patch([0 0 1 1-e 0+e 0+e],[0 1 1 1-e 1-e 0+e],c3);plot([0 1 1 0 0],[0 0 1 1 0]);
  wires:
  "p{1}"/1 -> Delays 1/1("p{1}")
  Delays 1/1("pd{1,1}") -> "IW{1,1}"/1("pd{1,1}")
  "IW{1,1}"/1("iz{1,1}") -> netsum/1
  "b{1}"/1 -> netsum/2
  netsum/1 -> tansig/1
  tansig/1 -> "a{1}"/1

== system ur10_NN_v1/QP-ECBF/Parameter Prediction/Layer 2 ==
  "a{1} " : Inport  PortDimensions=20
      mask Display: e = 0.06;c1 = [120 230 180]/255;c2 = ([120 230 180]+0)/(256+128);c3 = ([120 230 180]+128)/(256+128);patch([0 1 1 0],[0 0 1 1],c1);patch([0 1 1 1-e 1-e 0+e],[0 0 1 1-e 0+e 0+e],c2);patch([0 0 1 1-e 0+e 0+e],[0 1 1 1-e 1-e 0+e],c3);plot([0 1 1 0 0],[0 0 1 1 0]);
  Delays 1 : Subsystem
      mask Display: e = 0.06;c1 = [120 150 230]/255;c2 = ([120 150 230]+0)/383;c3 = ([120 150 230]+128)/383;patch([0 1 1 0],[0 0 1 1],c1);patch([0 1 1 1-e 1-e 0+e],[0 0 1 1-e 0+e 0+e],c2);patch([0 0 1 1-e 0+e 0+e],[0 1 1 1-e 1-e 0+e],c3);plot([0 1 1 0 0],[0 0 1 1 0]);disp('0');
  "LW{2,1}" : Subsystem
      mask Display: e = 0.06;c1 = [120 150 230]/255;c2 = ([120 150 230]+0)/383;c3 = ([120 150 230]+128)/383;patch([0 1 1 0],[0 0 1 1],c1);patch([0 1 1 1-e 1-e 0+e],[0 0 1 1-e 0+e 0+e],c2);patch([0 0 1 1-e 0+e 0+e],[0 1 1 1-e 1-e 0+e],c3);plot([0 1 1 0 0],[0 0 1 1 0]);disp('W');
  "b{2}" : Constant  Value=[0.0313188629546082564214515286948881112039089202880859375;0.1792620669296504931633506885191309265792369842529296875]
      mask Display: e = 0.06;c1 = [120 150 230]/255;c2 = ([120 150 230]+0)/383;c3 = ([120 150 230]+128)/383;patch([0 1 1 0],[0 0 1 1],c1);patch([0 1 1 1-e 1-e 0+e],[0 0 1 1-e 0+e 0+e],c2);patch([0 0 1 1-e 0+e 0+e],[0 1 1 1-e 1-e 0+e],c3);plot([0 1 1 0 0],[0 0 1 1 0]);disp('b');
  netsum : Sum  Inputs=2  InputSameDT=on  SaturateOnIntegerOverflow=on  OutDataTypeStr=Inherit: Same as first input
      mask Display: e = 0.06;c1 = [120 150 230]/255;c2 = ([120 150 230]+0)/383;c3 = ([120 150 230]+128)/383;patch([0 1 1 0],[0 0 1 1],c1);patch([0 1 1 1-e 1-e 0+e],[0 0 1 1-e 0+e 0+e],c2);patch([0 0 1 1-e 0+e 0+e],[0 1 1 1-e 1-e 0+e],c3);plot([0 1 1 0 0],[0 0 1 1 0]);disp('+');
  purelin : neural/Transfer Functions/purelin
  "a{2}" : Outport  InitialOutput=[0;0]
      mask Display: e = 0.06;c1 = [120 230 180]/255;c2 = ([120 230 180]+0)/(256+128);c3 = ([120 230 180]+128)/(256+128);patch([0 1 1 0],[0 0 1 1],c1);patch([0 1 1 1-e 1-e 0+e],[0 0 1 1-e 0+e 0+e],c2);patch([0 0 1 1-e 0+e 0+e],[0 1 1 1-e 1-e 0+e],c3);plot([0 1 1 0 0],[0 0 1 1 0]);
  wires:
  "a{1} "/1 -> Delays 1/1("p{2}")
  Delays 1/1("pd{2,1}") -> "LW{2,1}"/1("ad{2,1}")
  "LW{2,1}"/1("lz{2,1}") -> netsum/1
  "b{2}"/1 -> netsum/2
  netsum/1 -> purelin/1
  purelin/1 -> "a{2}"/1

== system ur10_NN_v1/QP-ECBF/Parameter Prediction/Process Input 1 ==
  x : Inport  PortDimensions=1
      mask Display: e = 0.06;c1 = [120 230 180]/255;c2 = ([120 230 180]+0)/(256+128);c3 = ([120 230 180]+128)/(256+128);patch([0 1 1 0],[0 0 1 1],c1);patch([0 1 1 1-e 1-e 0+e],[0 0 1 1-e 0+e 0+e],c2);patch([0 0 1 1-e 0+e 0+e],[0 1 1 1-e 1-e 0+e],c3);plot([0 1 1 0 0],[0 0 1 1 0]);
  mapminmax : neural/Processing Functions/mapminmax  xmin=0.0500000000000000027755575615629  xmax=0.299999999999999988897769753748  ymin=-1  ymax=1
  p : Outport  PortDimensions=1
      mask Display: e = 0.06;c1 = [120 230 180]/255;c2 = ([120 230 180]+0)/(256+128);c3 = ([120 230 180]+128)/(256+128);patch([0 1 1 0],[0 0 1 1],c1);patch([0 1 1 1-e 1-e 0+e],[0 0 1 1-e 0+e 0+e],c2);patch([0 0 1 1-e 0+e 0+e],[0 1 1 1-e 1-e 0+e],c3);plot([0 1 1 0 0],[0 0 1 1 0]);
  wires:
  x/1 -> mapminmax/1
  mapminmax/1 -> p/1

== system ur10_NN_v1/QP-ECBF/Parameter Prediction/Process Output 1 ==
  a : Inport  PortDimensions=2
      mask Display: e = 0.06;c1 = [120 230 180]/255;c2 = ([120 230 180]+0)/(256+128);c3 = ([120 230 180]+128)/(256+128);patch([0 1 1 0],[0 0 1 1],c1);patch([0 1 1 1-e 1-e 0+e],[0 0 1 1-e 0+e 0+e],c2);patch([0 0 1 1-e 0+e 0+e],[0 1 1 1-e 1-e 0+e],c3);plot([0 1 1 0 0],[0 0 1 1 0]);
  mapminmax_reverse : neural/Processing Functions/mapminmax_reverse  xmin=[3;3]  xmax=[100;100]  ymin=-1  ymax=1
  removeconstantrows_reverse : neural/Processing Functions/removeconstantrows_reverse  inputSize=3  constants=0.05  rearrange=[1 2 3]
  y : Outport  PortDimensions=3
      mask Display: e = 0.06;c1 = [120 230 180]/255;c2 = ([120 230 180]+0)/(256+128);c3 = ([120 230 180]+128)/(256+128);patch([0 1 1 0],[0 0 1 1],c1);patch([0 1 1 1-e 1-e 0+e],[0 0 1 1-e 0+e 0+e],c2);patch([0 0 1 1-e 0+e 0+e],[0 1 1 1-e 1-e 0+e],c3);plot([0 1 1 0 0],[0 0 1 1 0]);
  wires:
  a/1 -> mapminmax_reverse/1
  mapminmax_reverse/1 -> removeconstantrows_reverse/1
  removeconstantrows_reverse/1 -> y/1

== system ur10_NN_v1/QP-ECBF/Parameter Prediction/Layer 1/Delays 1 ==
  "p{1}" : Inport  PortDimensions=1
      mask Display: e = 0.06;c1 = [120 230 180]/255;c2 = ([120 230 180]+0)/(256+128);c3 = ([120 230 180]+128)/(256+128);patch([0 1 1 0],[0 0 1 1],c1);patch([0 1 1 1-e 1-e 0+e],[0 0 1 1-e 0+e 0+e],c2);patch([0 0 1 1-e 0+e 0+e],[0 1 1 1-e 1-e 0+e],c3);plot([0 1 1 0 0],[0 0 1 1 0]);
  mux : Mux  Inputs=1
      mask Display: e = 0.06;c1 = [120 150 230]/255;c2 = ([120 150 230]+0)/383;c3 = ([120 150 230]+128)/383;patch([0 1 1 0],[0 0 1 1],c1);patch([0 1 1 1-e 1-e 0+e],[0 0 1 1-e 0+e 0+e],c2);patch([0 0 1 1-e 0+e 0+e],[0 1 1 1-e 1-e 0+e],c3);plot([0 1 1 0 0],[0 0 1 1 0]);disp('Mux')
  "pd{1,1}" : Outport
      mask Display: e = 0.06;c1 = [120 230 180]/255;c2 = ([120 230 180]+0)/(256+128);c3 = ([120 230 180]+128)/(256+128);patch([0 1 1 0],[0 0 1 1],c1);patch([0 1 1 1-e 1-e 0+e],[0 0 1 1-e 0+e 0+e],c2);patch([0 0 1 1-e 0+e 0+e],[0 1 1 1-e 1-e 0+e],c3);plot([0 1 1 0 0],[0 0 1 1 0]);
  wires:
  "p{1}"/1 -> mux/1
  mux/1 -> "pd{1,1}"/1
